simulink model "Weltmodell"  (R2025b)
settings: Solver=VariableStepAuto  StartTime=0.0  StopTime=10.0  RelTol=1e-3
settings Model: DataDictionary=Weltmodell_dict.sldd  Creator=P28500  LastModifiedBy=P28500

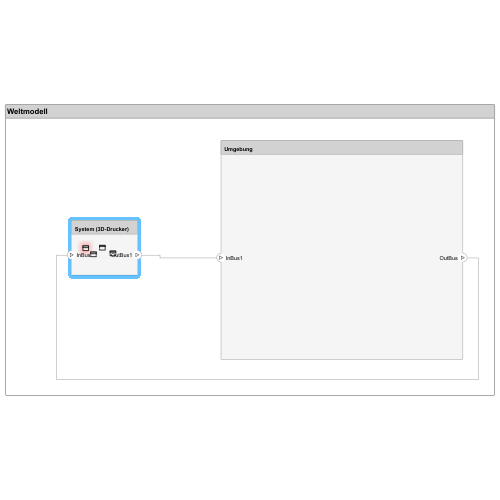
[thumbnail: Simulink's stored preview of the top-level diagram]
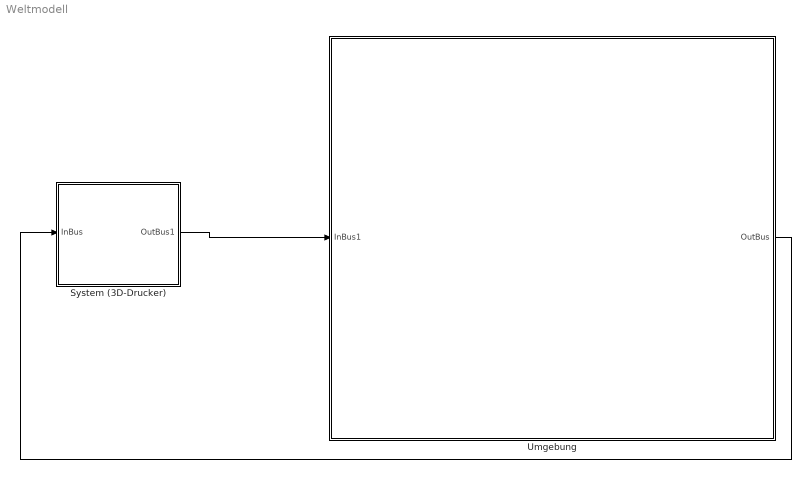
== system Weltmodell ==
  System (3D-Drucker) : Subsystem
      settings: PortSchema="{\"entries\":[{\"content\":{\"headerSize\":26,\"margin\":15,\"minimumSpacing\":25,\"sides\":[{\"content\":{\"connectorIds\":[\"In1\"]},\"type\":\"ConnectorPlacement.EquallySpacedRectSide\",\"uuid\":\"adede219-88a1-43e3-a9ee-c7f70639cd5e\"},{\"content\":{\"connectorIds\":[\"Out1\"],\"side\":\"RIGHT\"},\"type\":\"ConnectorPlacement.EquallySpacedRectSide\",\"uuid\":\"fed83cca-cd27-4665-ba9f-8e52d49a9f48\"},{\"content\":{\"side\":\"TOP\"},\"type\":\"ConnectorPlacement.EquallySpacedRectSide\",\"uuid\":\"78f760cc-fb79-4769-b611-1caac5772b0e\"}]},\"type\":\"ConnectorPlacement.EquallySpacedConnector\",\"uuid\":\"8c832b78-18d3-42e1-a909-b9e4105225d2\"}],\"packageUris\":[\"http://schema.mathworks.com/mf0/Connector/R2020b\"],\"version\":\"1.0\"}"
  Umgebung : Subsystem
      settings: PortSchema="{\"entries\":[{\"content\":{\"headerSize\":26,\"margin\":15,\"minimumSpacing\":25,\"sides\":[{\"content\":{\"connectorIds\":[\"In1\"]},\"type\":\"ConnectorPlacement.EquallySpacedRectSide\",\"uuid\":\"adede219-88a1-43e3-a9ee-c7f70639cd5e\"},{\"content\":{\"connectorIds\":[\"Out1\"],\"side\":\"RIGHT\"},\"type\":\"ConnectorPlacement.EquallySpacedRectSide\",\"uuid\":\"fed83cca-cd27-4665-ba9f-8e52d49a9f48\"},{\"content\":{\"side\":\"TOP\"},\"type\":\"ConnectorPlacement.EquallySpacedRectSide\",\"uuid\":\"78f760cc-fb79-4769-b611-1caac5772b0e\"}]},\"type\":\"ConnectorPlacement.EquallySpacedConnector\",\"uuid\":\"8c832b78-18d3-42e1-a909-b9e4105225d2\"}],\"packageUris\":[\"http://schema.mathworks.com/mf0/Connector/R2020b\"],\"version\":\"1.0\"}"
  wires:
  System (3D-Drucker)/1(OutBus1) -> Umgebung/1(InBus1)
  Umgebung/1(OutBus) -> System (3D-Drucker)/1(InBus)

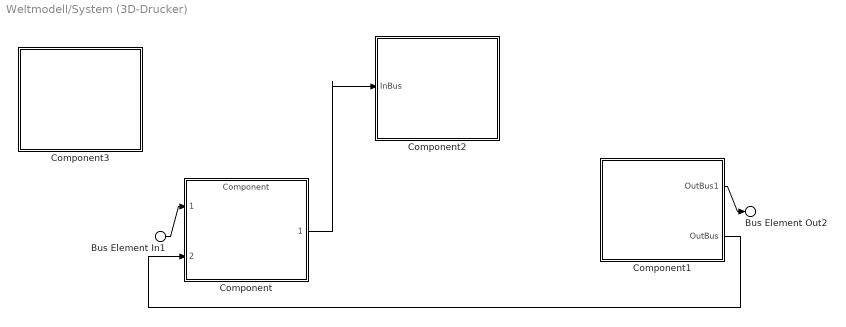
== system Weltmodell/System (3D-Drucker) ==
  Bus Element In1 : Inport  PortName=InBus
  Component : ModelReference  ModelNameDialog=Component  SimulationMode=Normal  ModelReferenceVersion=1.6
      settings: PortSchema="{\"entries\":[{\"content\":{\"headerSize\":38,\"margin\":15,\"minimumSpacing\":25,\"sides\":[{\"content\":{\"connectorIds\":[\"In1\",\"In2\"]},\"type\":\"ConnectorPlacement.EquallySpacedRectSide\",\"uuid\":\"adede219-88a1-43e3-a9ee-c7f70639cd5e\"},{\"content\":{\"connectorIds\":[\"Out1\"],\"side\":\"RIGHT\"},\"type\":\"ConnectorPlacement.EquallySpacedRectSide\",\"uuid\":\"fed83cca-cd27-4665-ba9f-8e52d49a9f48\"},{\"content\":{\"side\":\"TOP\"},\"type\":\"ConnectorPlacement.EquallySpacedRectSide\",\"uuid\":\"78f760cc-fb79-4769-b611-1caac5772b0e\"}]},\"type\":\"ConnectorPlacement.EquallySpacedConnector\",\"uuid\":\"8c832b78-18d3-42e1-a909-b9e4105225d2\"}],\"packageUris\":[\"http://schema.mathworks.com/mf0/Connector/R2020b\"],\"version\":\"1.0\"}"
  Component1 : Subsystem
      settings: PortSchema="{\"entries\":[{\"content\":{\"headerSize\":26,\"margin\":15,\"minimumSpacing\":25,\"sides\":[{\"content\":{},\"type\":\"ConnectorPlacement.EquallySpacedRectSide\",\"uuid\":\"adede219-88a1-43e3-a9ee-c7f70639cd5e\"},{\"content\":{\"connectorIds\":[\"Out1\",\"Out2\"],\"side\":\"RIGHT\"},\"type\":\"ConnectorPlacement.EquallySpacedRectSide\",\"uuid\":\"fed83cca-cd27-4665-ba9f-8e52d49a9f48\"},{\"content\":{\"side\":\"TOP\"},\"type\":\"ConnectorPlacement.EquallySpacedRectSide\",\"uuid\":\"78f760cc-fb79-4769-b611-1caac5772b0e\"}]},\"type\":\"ConnectorPlacement.EquallySpacedConnector\",\"uuid\":\"8c832b78-18d3-42e1-a909-b9e4105225d2\"}],\"packageUris\":[\"http://schema.mathworks.com/mf0/Connector/R2020b\"],\"version\":\"1.0\"}"
  Component2 : Stateflow chart  TreatAsAtomicUnit=on
      settings: PortSchema="{\"entries\":[{\"content\":{\"headerSize\":26,\"margin\":15,\"minimumSpacing\":25,\"sides\":[{\"content\":{\"connectorIds\":[\"In1\"]},\"type\":\"ConnectorPlacement.EquallySpacedRectSide\",\"uuid\":\"adede219-88a1-43e3-a9ee-c7f70639cd5e\"},{\"content\":{\"side\":\"RIGHT\"},\"type\":\"ConnectorPlacement.EquallySpacedRectSide\",\"uuid\":\"fed83cca-cd27-4665-ba9f-8e52d49a9f48\"},{\"content\":{\"side\":\"TOP\"},\"type\":\"ConnectorPlacement.EquallySpacedRectSide\",\"uuid\":\"78f760cc-fb79-4769-b611-1caac5772b0e\"}]},\"type\":\"ConnectorPlacement.EquallySpacedConnector\",\"uuid\":\"8c832b78-18d3-42e1-a909-b9e4105225d2\"}],\"packageUris\":[\"http://schema.mathworks.com/mf0/Connector/R2020b\"],\"version\":\"1.0\"}"
  Component3 : ModelReference  SimulationMode=Normal
      settings: PortSchema="{\"entries\":[{\"content\":{\"headerSize\":38,\"margin\":15,\"minimumSpacing\":25,\"sides\":[{\"content\":{},\"type\":\"ConnectorPlacement.EquallySpacedRectSide\",\"uuid\":\"2b37268d-e234-4367-98fd-6a080a1c3634\"},{\"content\":{\"side\":\"RIGHT\"},\"type\":\"ConnectorPlacement.EquallySpacedRectSide\",\"uuid\":\"ac6dfa5b-820e-4078-8e42-9d0e414b7dbc\"},{\"content\":{\"side\":\"TOP\"},\"type\":\"ConnectorPlacement.EquallySpacedRectSide\",\"uuid\":\"8b3c7907-3479-4e12-8636-a7b3377f996b\"}]},\"type\":\"ConnectorPlacement.EquallySpacedConnector\",\"uuid\":\"cdde60af-c4ad-49c1-94e4-038bc12dec86\"}],\"packageUris\":[\"http://schema.mathworks.com/mf0/Connector/R2020b\"],\"version\":\"1.0\"}"
  Bus Element Out2 : Outport  PortName=OutBus1
  wires:
  Component1/1(OutBus1) -> Bus Element Out2/1
  Component1/2(OutBus) -> Component/2
  Bus Element In1/1 -> Component/1
  Component/1 -> Component2/1(InBus)

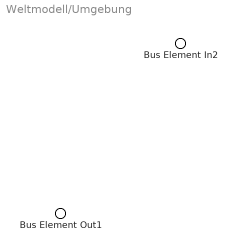
== system Weltmodell/Umgebung ==
  Bus Element In2 : Inport  PortName=InBus1
  Bus Element Out1 : Outport  PortName=OutBus

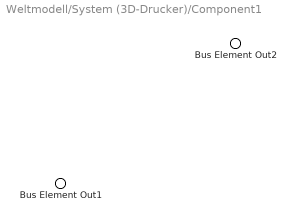
== system Weltmodell/System (3D-Drucker)/Component1 ==
  Bus Element Out2 : Outport  PortName=OutBus1
  Bus Element Out1 : Outport  Port=2  PortName=OutBus

== stateflow chart Weltmodell/System (3D-Drucker)/Component2 ==
  state ?
  state ?
  (default) -> ?
  ? -> ?
  data: InBus input
